simulink model "URDF_XG_Robot_Arm_Urdf_Control_V3"  (R2023a)
settings: Solver=FixedStepAuto  StartTime=0.0  StopTime=20  FixedStep=0.001  RelTol=1e-3
values from neighbouring files (symbols this model uses):
  D_H = [ ... (first row only)    [robot_kinematics_sym_v3_0.m]    (also in robot_kinematics_sym_v3_0_verify.m; robot_run.m)
undefined symbols (not defined in the file or in its folder): X, Y, Z
libraries: sm_lib x62, nesl_utility x11
(part 2 of 2)

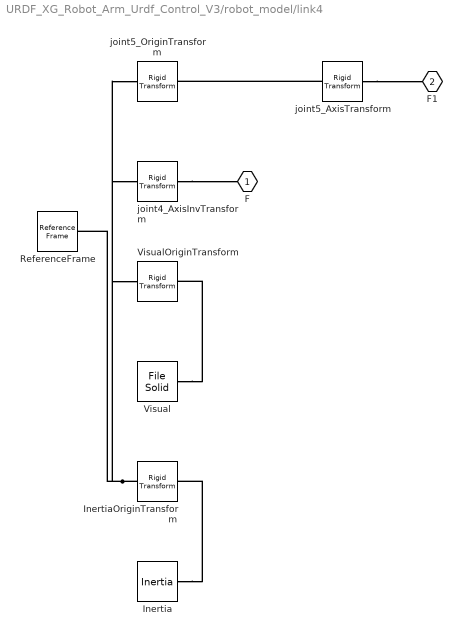
== system URDF_XG_Robot_Arm_Urdf_Control_V3/robot_model/link4 ==
  Inertia : sm_lib/Body Elements/Inertia  InertiaType=Custom  Mass=0.178465854809275  MassUnits=kg  CenterOfMass=[0, 0, 0]  CenterOfMassUnits=m  MomentsOfInertia=[0.00010542070955742, 0.000111293192127703, 4.4231117465552e-05]  MomentsOfInertiaUnits=kg*m^2  ProductsOfInertia=[-4.12005754357462e-07, -1.17627516604833e-07, -1.56493108731347e-07]  ProductsOfInertiaUnits=kg*m^2  GraphicType=None  MarkerShape=Inertia  MarkerSize=20  GraphicVisPropType=SimpleVisualProperties  GraphicDiffuseColor=[0.5 0.5 0.5]  GraphicSpecularColor=[0.5 0.5 0.5 1.0]  GraphicAmbientColor=[0.15 0.15 0.15 1.0]  GraphicEmissiveColor=[0.0 0.0 0.0 1.0]  GraphicShininess=75  GraphicOpacity=1.0
  InertiaOriginTransform : sm_lib/Frames and Transforms/Rigid Transform  TranslationMethod=Cartesian  TranslationStandardOffset=0  TranslationStandardOffsetUnits=m  TranslationStandardAxis=+Z  TranslationCartesianOffset=[-2.8160808468243e-05, -0.00682767077230628, 0.0299455082197141]  TranslationCartesianOffsetUnits=m  TranslationROffset=0  TranslationROffsetUnits=m  TranslationZOffset=0  TranslationZOffsetUnits=m  TranslationThetaOffset=0  TranslationThetaOffsetUnits=deg  RotationMethod=RotationSequence  RotationAngleUnits=deg  RotationStandardAxis=+Z  RotationAngle=0.0  RotationArbitraryAxis=[0 0 1]  FollAlignAxisA=+X  BaseAlignAxisA=+Y  FollAlignAxisB=+Y  BaseAlignAxisB=+Z  RotationSequenceAxes=BaseAxes  RotationSequence=XYZ  RotationSequenceAngles=[0, 0, 0]  RotationSequenceAnglesUnits=rad  RotationMatrix=[1 0 0; 0 1 0; 0 0 1]  Quaternion=[1 0 0 0]
  ReferenceFrame : sm_lib/Frames and Transforms/Reference Frame
  Visual : sm_lib/Body Elements/File Solid  ExtGeomFileName=URDF_XG_Robot_Arm_Urdf_V1_1/meshes/link4.STL  UnitType=Custom  ExtGeomFileUnits=m  StepReaderType=HEX  ExportConvexHullGeometry=off  InertiaType=Custom  Mass=0  MassUnits=kg  CenterOfMass=[0, 0, 0]  CenterOfMassUnits=m  MomentsOfInertia=[0, 0, 0]  MomentsOfInertiaUnits=kg*m^2  ProductsOfInertia=[0, 0, 0]  ProductsOfInertiaUnits=kg*m^2  BasedOnType=DensityFromFile  Density=1000  DensityUnits=kg/m^3  DoExposeReferenceFrame=on  SerializedFrames=<Frames/>  GraphicType=FromGeometry  MarkerShape=Sphere  MarkerSize=10  GraphicVisPropType=SimpleVisualProperties  GraphicDiffuseColor=[0.752941176470588, 0.752941176470588, 0.752941176470588]  GraphicSpecularColor=[0.5 0.5 0.5 1.0]  GraphicAmbientColor=[0.15 0.15 0.15 1.0]  GraphicEmissiveColor=[0.0 0.0 0.0 1.0]  GraphicShininess=75  GraphicOpacity=1
  VisualOriginTransform : sm_lib/Frames and Transforms/Rigid Transform  TranslationMethod=Cartesian  TranslationStandardOffset=0  TranslationStandardOffsetUnits=m  TranslationStandardAxis=+Z  TranslationCartesianOffset=[0, 0, 0]  TranslationCartesianOffsetUnits=m  TranslationROffset=0  TranslationROffsetUnits=m  TranslationZOffset=0  TranslationZOffsetUnits=m  TranslationThetaOffset=0  TranslationThetaOffsetUnits=deg  RotationMethod=RotationSequence  RotationAngleUnits=deg  RotationStandardAxis=+Z  RotationAngle=0.0  RotationArbitraryAxis=[0 0 1]  FollAlignAxisA=+X  BaseAlignAxisA=+Y  FollAlignAxisB=+Y  BaseAlignAxisB=+Z  RotationSequenceAxes=BaseAxes  RotationSequence=XYZ  RotationSequenceAngles=[0, 0, 0]  RotationSequenceAnglesUnits=rad  RotationMatrix=[1 0 0; 0 1 0; 0 0 1]  Quaternion=[1 0 0 0]
  joint4_AxisInvTransform : sm_lib/Frames and Transforms/Rigid Transform  TranslationMethod=Cartesian  TranslationStandardOffset=0  TranslationStandardOffsetUnits=m  TranslationStandardAxis=+Z  TranslationCartesianOffset=[0, 0, 0]  TranslationCartesianOffsetUnits=m  TranslationROffset=0  TranslationROffsetUnits=m  TranslationZOffset=0  TranslationZOffsetUnits=m  TranslationThetaOffset=0  TranslationThetaOffsetUnits=deg  RotationMethod=ArbitraryAxis  RotationAngleUnits=rad  RotationStandardAxis=+Z  RotationAngle=0  RotationArbitraryAxis=[1, 0, 0]  FollAlignAxisA=+X  BaseAlignAxisA=+Y  FollAlignAxisB=+Y  BaseAlignAxisB=+Z  RotationSequenceAxes=FollowerAxes  RotationSequence=XYX  RotationSequenceAngles=[0 0 0]  RotationSequenceAnglesUnits=deg  RotationMatrix=[1 0 0; 0 1 0; 0 0 1]  Quaternion=[1 0 0 0]
  joint5_AxisTransform : sm_lib/Frames and Transforms/Rigid Transform  TranslationMethod=Cartesian  TranslationStandardOffset=0  TranslationStandardOffsetUnits=m  TranslationStandardAxis=+Z  TranslationCartesianOffset=[0, 0, 0]  TranslationCartesianOffsetUnits=m  TranslationROffset=0  TranslationROffsetUnits=m  TranslationZOffset=0  TranslationZOffsetUnits=m  TranslationThetaOffset=0  TranslationThetaOffsetUnits=deg  RotationMethod=ArbitraryAxis  RotationAngleUnits=rad  RotationStandardAxis=+Z  RotationAngle=0  RotationArbitraryAxis=[1, 0, 0]  FollAlignAxisA=+X  BaseAlignAxisA=+Y  FollAlignAxisB=+Y  BaseAlignAxisB=+Z  RotationSequenceAxes=FollowerAxes  RotationSequence=XYX  RotationSequenceAngles=[0 0 0]  RotationSequenceAnglesUnits=deg  RotationMatrix=[1 0 0; 0 1 0; 0 0 1]  Quaternion=[1 0 0 0]
  joint5_OriginTransform : sm_lib/Frames and Transforms/Rigid Transform  TranslationMethod=Cartesian  TranslationStandardOffset=0  TranslationStandardOffsetUnits=m  TranslationStandardAxis=+Z  TranslationCartesianOffset=[0, 0, 0]  TranslationCartesianOffsetUnits=m  TranslationROffset=0  TranslationROffsetUnits=m  TranslationZOffset=0  TranslationZOffsetUnits=m  TranslationThetaOffset=0  TranslationThetaOffsetUnits=deg  RotationMethod=RotationSequence  RotationAngleUnits=deg  RotationStandardAxis=+Z  RotationAngle=0.0  RotationArbitraryAxis=[0 0 1]  FollAlignAxisA=+X  BaseAlignAxisA=+Y  FollAlignAxisB=+Y  BaseAlignAxisB=+Z  RotationSequenceAxes=BaseAxes  RotationSequence=XYZ  RotationSequenceAngles=[1.5708, -1.5708, 0]  RotationSequenceAnglesUnits=rad  RotationMatrix=[1 0 0; 0 1 0; 0 0 1]  Quaternion=[1 0 0 0]
  F : PMIOPort  Side=Left
  F1 : PMIOPort  Port=2  Side=Right
  connections:
  Inertia/RConn1 -- InertiaOriginTransform/RConn1
  ReferenceFrame/RConn1 -- InertiaOriginTransform/LConn1 -- VisualOriginTransform/LConn1 -- joint4_AxisInvTransform/LConn1 -- joint5_OriginTransform/LConn1
  Visual/RConn1 -- VisualOriginTransform/RConn1
  joint4_AxisInvTransform/RConn1 -- F/RConn1
  joint5_AxisTransform/RConn1 -- F1/RConn1
  joint5_AxisTransform/LConn1 -- joint5_OriginTransform/RConn1

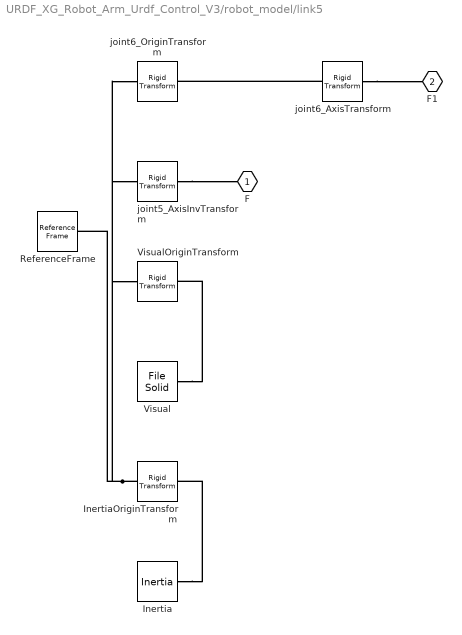
== system URDF_XG_Robot_Arm_Urdf_Control_V3/robot_model/link5 ==
  Inertia : sm_lib/Body Elements/Inertia  InertiaType=Custom  Mass=0.15793222447205  MassUnits=kg  CenterOfMass=[0, 0, 0]  CenterOfMassUnits=m  MomentsOfInertia=[0.000135933655838788, 5.60082572905534e-05, 0.000121456700565665]  MomentsOfInertiaUnits=kg*m^2  ProductsOfInertia=[3.96647905066164e-05, 8.388614449562571e-09, -6.33132038702403e-08]  ProductsOfInertiaUnits=kg*m^2  GraphicType=None  MarkerShape=Inertia  MarkerSize=20  GraphicVisPropType=SimpleVisualProperties  GraphicDiffuseColor=[0.5 0.5 0.5]  GraphicSpecularColor=[0.5 0.5 0.5 1.0]  GraphicAmbientColor=[0.15 0.15 0.15 1.0]  GraphicEmissiveColor=[0.0 0.0 0.0 1.0]  GraphicShininess=75  GraphicOpacity=1.0
  InertiaOriginTransform : sm_lib/Frames and Transforms/Rigid Transform  TranslationMethod=Cartesian  TranslationStandardOffset=0  TranslationStandardOffsetUnits=m  TranslationStandardAxis=+Z  TranslationCartesianOffset=[0.000156431818420899, -0.0617917966301206, -0.0100252833788212]  TranslationCartesianOffsetUnits=m  TranslationROffset=0  TranslationROffsetUnits=m  TranslationZOffset=0  TranslationZOffsetUnits=m  TranslationThetaOffset=0  TranslationThetaOffsetUnits=deg  RotationMethod=RotationSequence  RotationAngleUnits=deg  RotationStandardAxis=+Z  RotationAngle=0.0  RotationArbitraryAxis=[0 0 1]  FollAlignAxisA=+X  BaseAlignAxisA=+Y  FollAlignAxisB=+Y  BaseAlignAxisB=+Z  RotationSequenceAxes=BaseAxes  RotationSequence=XYZ  RotationSequenceAngles=[0, 0, 0]  RotationSequenceAnglesUnits=rad  RotationMatrix=[1 0 0; 0 1 0; 0 0 1]  Quaternion=[1 0 0 0]
  ReferenceFrame : sm_lib/Frames and Transforms/Reference Frame
  Visual : sm_lib/Body Elements/File Solid  ExtGeomFileName=URDF_XG_Robot_Arm_Urdf_V1_1/meshes/link5.STL  UnitType=Custom  ExtGeomFileUnits=m  StepReaderType=HEX  ExportConvexHullGeometry=off  InertiaType=Custom  Mass=0  MassUnits=kg  CenterOfMass=[0, 0, 0]  CenterOfMassUnits=m  MomentsOfInertia=[0, 0, 0]  MomentsOfInertiaUnits=kg*m^2  ProductsOfInertia=[0, 0, 0]  ProductsOfInertiaUnits=kg*m^2  BasedOnType=DensityFromFile  Density=1000  DensityUnits=kg/m^3  DoExposeReferenceFrame=on  SerializedFrames=<Frames/>  GraphicType=FromGeometry  MarkerShape=Sphere  MarkerSize=10  GraphicVisPropType=SimpleVisualProperties  GraphicDiffuseColor=[0.752941176470588, 0.752941176470588, 0.752941176470588]  GraphicSpecularColor=[0.5 0.5 0.5 1.0]  GraphicAmbientColor=[0.15 0.15 0.15 1.0]  GraphicEmissiveColor=[0.0 0.0 0.0 1.0]  GraphicShininess=75  GraphicOpacity=1
  VisualOriginTransform : sm_lib/Frames and Transforms/Rigid Transform  TranslationMethod=Cartesian  TranslationStandardOffset=0  TranslationStandardOffsetUnits=m  TranslationStandardAxis=+Z  TranslationCartesianOffset=[0, 0, 0]  TranslationCartesianOffsetUnits=m  TranslationROffset=0  TranslationROffsetUnits=m  TranslationZOffset=0  TranslationZOffsetUnits=m  TranslationThetaOffset=0  TranslationThetaOffsetUnits=deg  RotationMethod=RotationSequence  RotationAngleUnits=deg  RotationStandardAxis=+Z  RotationAngle=0.0  RotationArbitraryAxis=[0 0 1]  FollAlignAxisA=+X  BaseAlignAxisA=+Y  FollAlignAxisB=+Y  BaseAlignAxisB=+Z  RotationSequenceAxes=BaseAxes  RotationSequence=XYZ  RotationSequenceAngles=[0, 0, 0]  RotationSequenceAnglesUnits=rad  RotationMatrix=[1 0 0; 0 1 0; 0 0 1]  Quaternion=[1 0 0 0]
  joint5_AxisInvTransform : sm_lib/Frames and Transforms/Rigid Transform  TranslationMethod=Cartesian  TranslationStandardOffset=0  TranslationStandardOffsetUnits=m  TranslationStandardAxis=+Z  TranslationCartesianOffset=[0, 0, 0]  TranslationCartesianOffsetUnits=m  TranslationROffset=0  TranslationROffsetUnits=m  TranslationZOffset=0  TranslationZOffsetUnits=m  TranslationThetaOffset=0  TranslationThetaOffsetUnits=deg  RotationMethod=ArbitraryAxis  RotationAngleUnits=rad  RotationStandardAxis=+Z  RotationAngle=0  RotationArbitraryAxis=[1, 0, 0]  FollAlignAxisA=+X  BaseAlignAxisA=+Y  FollAlignAxisB=+Y  BaseAlignAxisB=+Z  RotationSequenceAxes=FollowerAxes  RotationSequence=XYX  RotationSequenceAngles=[0 0 0]  RotationSequenceAnglesUnits=deg  RotationMatrix=[1 0 0; 0 1 0; 0 0 1]  Quaternion=[1 0 0 0]
  joint6_AxisTransform : sm_lib/Frames and Transforms/Rigid Transform  TranslationMethod=Cartesian  TranslationStandardOffset=0  TranslationStandardOffsetUnits=m  TranslationStandardAxis=+Z  TranslationCartesianOffset=[0, 0, 0]  TranslationCartesianOffsetUnits=m  TranslationROffset=0  TranslationROffsetUnits=m  TranslationZOffset=0  TranslationZOffsetUnits=m  TranslationThetaOffset=0  TranslationThetaOffsetUnits=deg  RotationMethod=ArbitraryAxis  RotationAngleUnits=rad  RotationStandardAxis=+Z  RotationAngle=0  RotationArbitraryAxis=[1, 0, 0]  FollAlignAxisA=+X  BaseAlignAxisA=+Y  FollAlignAxisB=+Y  BaseAlignAxisB=+Z  RotationSequenceAxes=FollowerAxes  RotationSequence=XYX  RotationSequenceAngles=[0 0 0]  RotationSequenceAnglesUnits=deg  RotationMatrix=[1 0 0; 0 1 0; 0 0 1]  Quaternion=[1 0 0 0]
  joint6_OriginTransform : sm_lib/Frames and Transforms/Rigid Transform  TranslationMethod=Cartesian  TranslationStandardOffset=0  TranslationStandardOffsetUnits=m  TranslationStandardAxis=+Z  TranslationCartesianOffset=[0, -0.125, 0]  TranslationCartesianOffsetUnits=m  TranslationROffset=0  TranslationROffsetUnits=m  TranslationZOffset=0  TranslationZOffsetUnits=m  TranslationThetaOffset=0  TranslationThetaOffsetUnits=deg  RotationMethod=RotationSequence  RotationAngleUnits=deg  RotationStandardAxis=+Z  RotationAngle=0.0  RotationArbitraryAxis=[0 0 1]  FollAlignAxisA=+X  BaseAlignAxisA=+Y  FollAlignAxisB=+Y  BaseAlignAxisB=+Z  RotationSequenceAxes=BaseAxes  RotationSequence=XYZ  RotationSequenceAngles=[1.5708, 0, 0]  RotationSequenceAnglesUnits=rad  RotationMatrix=[1 0 0; 0 1 0; 0 0 1]  Quaternion=[1 0 0 0]
  F : PMIOPort  Side=Left
  F1 : PMIOPort  Port=2  Side=Right
  connections:
  Inertia/RConn1 -- InertiaOriginTransform/RConn1
  ReferenceFrame/RConn1 -- InertiaOriginTransform/LConn1 -- VisualOriginTransform/LConn1 -- joint5_AxisInvTransform/LConn1 -- joint6_OriginTransform/LConn1
  Visual/RConn1 -- VisualOriginTransform/RConn1
  joint5_AxisInvTransform/RConn1 -- F/RConn1
  joint6_AxisTransform/RConn1 -- F1/RConn1
  joint6_AxisTransform/LConn1 -- joint6_OriginTransform/RConn1

== matlab function URDF_XG_Robot_Arm_Urdf_Control_V3/MATLAB Function1 ==
  data: thetas input; theta output; index input
function theta = theta_selection(thetas, index)

theta = thetas(index, :);

== matlab function URDF_XG_Robot_Arm_Urdf_Control_V3/inv_kinematic/MATLAB Function13 ==
  data: joint_thetas input; thetas_ret output
function thetas_ret = joint_rad2deg(joint_thetas)
thetas_ret = joint_thetas;
for i = 1:4
    for j = 1:6
        thetas_ret(i,j) = rad2deg(thetas_ret(i,j));
    end
end

== matlab function URDF_XG_Robot_Arm_Urdf_Control_V3/inv_kinematic/MATLAB Function1 ==
  data: T_target input; joint_thetas_ret output; joint_thetas input; D_H input
function joint_thetas_ret  = get_theta2(T_target, joint_thetas, D_H)
joint_thetas_ret = zeros(4,6);
joint_thetas_ret(1,:) = joint_thetas(1,:);
joint_thetas_ret(2,:) = joint_thetas(1,:);
joint_thetas_ret(3,:) = joint_thetas(2,:);
joint_thetas_ret(4,:) = joint_thetas(2,:);
joint_thetas_ret(1,2) = get_theta2_1(T_target, joint_thetas_ret(1,3), D_H);
joint_thetas_ret(2,2) = get_theta2_2(T_target, joint_thetas_ret(2,3), D_H);
joint_thetas_ret(3,2) = get_theta2_1(T_target, joint_thetas_ret(3,3), D_H);
joint_thetas_ret(4,2) = get_theta2_2(T_target, joint_thetas_ret(4,3), D_H);
end

function theta2_1 = get_theta2_1(T_target, theta3, D_H)
a_cow = D_H(:, 1);
d_cow = D_H(:, 3);
a2 = a_cow(3);
a3 = a_cow(4);
d4 = d_cow(4);
pz = T_target(3,4);
u1_theta2 = -(a2 + (a2^2 + 2*cos(theta3)*a2*a3 - 2*sin(theta3)*a2*d4 + a3^2 + d4^2 - pz^2)^(1/2) + a3*cos(theta3) - d4*sin(theta3))/(d4*cos(theta3) - pz + a3*sin(theta3));
theta2_1 = atan(u1_theta2)*2;
end

function theta2_2 = get_theta2_2(T_target, theta3, D_H)
a_cow = D_H(:, 1);
d_cow = D_H(:, 3);
a2 = a_cow(3);
a3 = a_cow(4);
d4 = d_cow(4);
pz = T_target(3,4);
u2_theta2 = -(a2 - (a2^2 + 2*cos(theta3)*a2*a3 - 2*sin(theta3)*a2*d4 + a3^2 + d4^2 - pz^2)^(1/2) + a3*cos(theta3) - d4*sin(theta3))/(d4*cos(theta3) - pz + a3*sin(theta3));
theta2_2 = atan(u2_theta2)*2;
end

== matlab function URDF_XG_Robot_Arm_Urdf_Control_V3/inv_kinematic/MATLAB Function ==
  data: T_target input; joint_theatas_ret output; D_H input
function joint_theatas_ret  = get_theta3(T_target, D_H)
a_cow = D_H(:, 1);
d_cow = D_H(:, 3);
a2 = a_cow(3);
a3 = a_cow(4);
d4 = d_cow(4);
px = T_target(1,4);
py = T_target(2,4);
pz = T_target(3,4);
joint_theatas_ret = zeros(2,6);

u1_theta3 = -(2*a2*d4 + (- a2^4 + 2*a2^2*a3^2 + 2*a2^2*d4^2 + 2*a2^2*px^2 + 2*a2^2*py^2 + 2*a2^2*pz^2 - a3^4 - 2*a3^2*d4^2 + 2*a3^2*px^2 + 2*a3^2*py^2 + 2*a3^2*pz^2 - d4^4 + 2*d4^2*px^2 + 2*d4^2*py^2 + 2*d4^2*pz^2 - px^4 - 2*px^2*py^2 - 2*px^2*pz^2 - py^4 - 2*py^2*pz^2 - pz^4)^(1/2))/(- a2^2 + 2*a2*a3 - a3^2 - d4^2 + px^2 + py^2 + pz^2);
u2_theta3 = -(2*a2*d4 - (- a2^4 + 2*a2^2*a3^2 + 2*a2^2*d4^2 + 2*a2^2*px^2 + 2*a2^2*py^2 + 2*a2^2*pz^2 - a3^4 - 2*a3^2*d4^2 + 2*a3^2*px^2 + 2*a3^2*py^2 + 2*a3^2*pz^2 - d4^4 + 2*d4^2*px^2 + 2*d4^2*py^2 + 2*d4^2*pz^2 - px^4 - 2*px^2*py^2 - 2*px^2*pz^2 - py^4 - 2*py^2*pz^2 - pz^4)^(1/2))/(- a2^2 + 2*a2*a3 - a3^2 - d4^2 + px^2 + py^2 + pz^2);
theta3_1 = atan(u1_theta3)*2;
theta3_2 = atan(u2_theta3)*2;
joint_theatas_ret(1, 3) = theta3_1;
joint_theatas_ret(2, 3) = theta3_2;
end

== matlab function URDF_XG_Robot_Arm_Urdf_Control_V3/inv_kinematic/MATLAB Function2 ==
  data: T_target input; joint_thetas output; joint_thetas input; D_H input
function joint_thetas  = get_theta1(T_target, joint_thetas, D_H)
joint_thetas(1,1) = get_theta1_(T_target, joint_thetas(1,:), D_H);
joint_thetas(2,1) = get_theta1_(T_target, joint_thetas(2,:), D_H);
joint_thetas(3,1) = get_theta1_(T_target, joint_thetas(3,:), D_H);
joint_thetas(4,1) = get_theta1_(T_target, joint_thetas(4,:), D_H);
end

function theta1_1 = get_theta1_(T_target, thetas, D_H)
a_cow = D_H(:, 1);
d_cow = D_H(:, 3);
a2 = a_cow(3);
a3 = a_cow(4);
d4 = d_cow(4);
px = T_target(1,4);
py = T_target(2,4);
pz = T_target(3,4);

theta2 = thetas(2);
theta3 = thetas(3);

v1 = (cos(theta2)*(a2 + a3*cos(theta3) - d4*sin(theta3)) + sin(theta2)*(d4*cos(theta3) + a3*sin(theta3)));
v2 = -px/v1;

% 设置容忍度
tolerance = 1e-4;

u1_theta1 = ((v2+1)/(1-v2))^(1/2);
if abs(py - (2*u1_theta1*v1)/(u1_theta1^2 + 1)) > tolerance
    u1_theta1 = -u1_theta1;
end
theta1_1 = atan(u1_theta1)*2;
end

== matlab function URDF_XG_Robot_Arm_Urdf_Control_V3/inv_kinematic/MATLAB Function3 ==
  data: T_target input; joint_thetas_ret output; joint_thetas input; D_H input
function joint_thetas_ret  = get_theta5(T_target, joint_thetas, D_H)
joint_thetas_ret = joint_thetas;
for i = 1:4
    joint_thetas_ret(i, 5) = get_theta5_(T_target, joint_thetas_ret(i, :), D_H);
end
end

function theta5 = get_theta5_(T_target, thetas, D_H)
a_cow = D_H(:, 1);
d_cow = D_H(:, 3);
a2 = a_cow(3);
a3 = a_cow(4);
d4 = d_cow(4);
px = T_target(1,4);
py = T_target(2,4);
pz = T_target(3,4);
nx = T_target(1,1);
ny = T_target(2,1);
nz = T_target(3,1);
ox = T_target(1,2);
oy = T_target(2,2);
oz = T_target(3,2);
ax= T_target(1,3);
ay= T_target(2,3);
az= T_target(3,3);
theta2 = thetas(2);
theta3 = thetas(3);
theta1 = thetas(1);

r32 = - (oz*(cos(theta2)*cos(theta3) + sin(theta2)*sin(theta3)))/(cos(theta2)^2*cos(theta3)^2 + cos(theta2)^2*sin(theta3)^2 + cos(theta3)^2*sin(theta2)^2 + sin(theta2)^2*sin(theta3)^2) - (ox*(cos(theta1)*cos(theta2)*sin(theta3) - cos(theta1)*cos(theta3)*sin(theta2)))/(cos(theta1)^2*cos(theta2)^2*cos(theta3)^2 + cos(theta1)^2*cos(theta2)^2*sin(theta3)^2 + cos(theta1)^2*cos(theta3)^2*sin(theta2)^2 + cos(theta1)^2*sin(theta2)^2*sin(theta3)^2 + cos(theta2)^2*cos(theta3)^2*sin(theta1)^2 + cos(theta2)^2*sin(theta1)^2*sin(theta3)^2 + cos(theta3)^2*sin(theta1)^2*sin(theta2)^2 + sin(theta1)^2*sin(theta2)^2*sin(theta3)^2) - (oy*(cos(theta2)*sin(theta1)*sin(theta3) - cos(theta3)*sin(theta1)*sin(theta2)))/(cos(theta1)^2*cos(theta2)^2*cos(theta3)^2 + cos(theta1)^2*cos(theta2)^2*sin(theta3)^2 + cos(theta1)^2*cos(theta3)^2*sin(theta2)^2 + cos(theta1)^2*sin(theta2)^2*sin(theta3)^2 + cos(theta2)^2*cos(theta3)^2*sin(theta1)^2 + cos(theta2)^2*sin(theta1)^2*sin(theta3)^2 + cos(theta3)^2*sin(theta1)^2*sin(theta2)^2 + sin(theta1)^2*sin(theta2)^2*sin(theta3)^2);
r31 = - (nz*(cos(theta2)*cos(theta3) + sin(theta2)*sin(theta3)))/(cos(theta2)^2*cos(theta3)^2 + cos(theta2)^2*sin(theta3)^2 + cos(theta3)^2*sin(theta2)^2 + sin(theta2)^2*sin(theta3)^2) - (nx*(cos(theta1)*cos(theta2)*sin(theta3) - cos(theta1)*cos(theta3)*sin(theta2)))/(cos(theta1)^2*cos(theta2)^2*cos(theta3)^2 + cos(theta1)^2*cos(theta2)^2*sin(theta3)^2 + cos(theta1)^2*cos(theta3)^2*sin(theta2)^2 + cos(theta1)^2*sin(theta2)^2*sin(theta3)^2 + cos(theta2)^2*cos(theta3)^2*sin(theta1)^2 + cos(theta2)^2*sin(theta1)^2*sin(theta3)^2 + cos(theta3)^2*sin(theta1)^2*sin(theta2)^2 + sin(theta1)^2*sin(theta2)^2*sin(theta3)^2) - (ny*(cos(theta2)*sin(theta1)*sin(theta3) - cos(theta3)*sin(theta1)*sin(theta2)))/(cos(theta1)^2*cos(theta2)^2*cos(theta3)^2 + cos(theta1)^2*cos(theta2)^2*sin(theta3)^2 + cos(theta1)^2*cos(theta3)^2*sin(theta2)^2 + cos(theta1)^2*sin(theta2)^2*sin(theta3)^2 + cos(theta2)^2*cos(theta3)^2*sin(theta1)^2 + cos(theta2)^2*sin(theta1)^2*sin(theta3)^2 + cos(theta3)^2*sin(theta1)^2*sin(theta2)^2 + sin(theta1)^2*sin(theta2)^2*sin(theta3)^2);
r33 = - (az*(cos(theta2)*cos(theta3) + sin(theta2)*sin(theta3)))/(cos(theta2)^2*cos(theta3)^2 + cos(theta2)^2*sin(theta3)^2 + cos(theta3)^2*sin(theta2)^2 + sin(theta2)^2*sin(theta3)^2) - (ax*(cos(theta1)*cos(theta2)*sin(theta3) - cos(theta1)*cos(theta3)*sin(theta2)))/(cos(theta1)^2*cos(theta2)^2*cos(theta3)^2 + cos(theta1)^2*cos(theta2)^2*sin(theta3)^2 + cos(theta1)^2*cos(theta3)^2*sin(theta2)^2 + cos(theta1)^2*sin(theta2)^2*sin(theta3)^2 + cos(theta2)^2*cos(theta3)^2*sin(theta1)^2 + cos(theta2)^2*sin(theta1)^2*sin(theta3)^2 + cos(theta3)^2*sin(theta1)^2*sin(theta2)^2 + sin(theta1)^2*sin(theta2)^2*sin(theta3)^2) - (ay*(cos(theta2)*sin(theta1)*sin(theta3) - cos(theta3)*sin(theta1)*sin(theta2)))/(cos(theta1)^2*cos(theta2)^2*cos(theta3)^2 + cos(theta1)^2*cos(theta2)^2*sin(theta3)^2 + cos(theta1)^2*cos(theta3)^2*sin(theta2)^2 + cos(theta1)^2*sin(theta2)^2*sin(theta3)^2 + cos(theta2)^2*cos(theta3)^2*sin(theta1)^2 + cos(theta2)^2*sin(theta1)^2*sin(theta3)^2 + cos(theta3)^2*sin(theta1)^2*sin(theta2)^2 + sin(theta1)^2*sin(theta2)^2*sin(theta3)^2);
theta5 = atan2(sqrt(r32^2 + r31^2), r33);
theta5 = -theta5 + pi;
end

== matlab function URDF_XG_Robot_Arm_Urdf_Control_V3/inv_kinematic/MATLAB Function4 ==
  data: T_target input; joint_thetas_ret output; joint_thetas input; D_H input
function joint_thetas_ret  = get_theta4(T_target, joint_thetas, D_H)
joint_thetas_ret = joint_thetas;
for i = 1:4
    joint_thetas_ret(i, 4) = get_theta4_(T_target, joint_thetas_ret(i, :), D_H);
end
end

function theta4_value = get_theta4_(T_target, thetas, D_H)
% deg_theta5_zyz = rad2deg(-thetas(5) + pi);
% if deg_theta5_zyz == 0 || deg_theta5_zyz == 180
%     theta4_value = 0;
%     return;
% end
a_cow = D_H(:, 1);
d_cow = D_H(:, 3);
a2 = a_cow(3);
a3 = a_cow(4);
d4 = d_cow(4);
px = T_target(1,4);
py = T_target(2,4);
pz = T_target(3,4);
nx = T_target(1,1);
ny = T_target(2,1);
nz = T_target(3,1);
ox = T_target(1,2);
oy = T_target(2,2);
oz = T_target(3,2);
ax= T_target(1,3);
ay= T_target(2,3);
az= T_target(3,3);
theta2 = thetas(2);
theta3 = thetas(3);
theta1 = thetas(1);
theta4 = 0; % 这里特殊，用于坐标系对齐
r23 = -(ax*cos(theta1)*cos(theta2)*cos(theta3)*sin(theta4) - ax*cos(theta4)*sin(theta1)*sin(theta2)^2*sin(theta3)^2 + ay*cos(theta2)*cos(theta3)*sin(theta1)*sin(theta4) + ax*cos(theta1)*sin(theta2)*sin(theta3)*sin(theta4) + ay*sin(theta1)*sin(theta2)*sin(theta3)*sin(theta4) - az*cos(theta1)^2*cos(theta2)*sin(theta3)*sin(theta4) + az*cos(theta1)^2*cos(theta3)*sin(theta2)*sin(theta4) - az*cos(theta2)*sin(theta1)^2*sin(theta3)*sin(theta4) + az*cos(theta3)*sin(theta1)^2*sin(theta2)*sin(theta4) + ay*cos(theta1)*cos(theta2)^2*cos(theta3)^2*cos(theta4) - ax*cos(theta2)^2*cos(theta3)^2*cos(theta4)*sin(theta1) + ay*cos(theta1)*cos(theta2)^2*cos(theta4)*sin(theta3)^2 + ay*cos(theta1)*cos(theta3)^2*cos(theta4)*sin(theta2)^2 - ax*cos(theta2)^2*cos(theta4)*sin(theta1)*sin(theta3)^2 - ax*cos(theta3)^2*cos(theta4)*sin(theta1)*sin(theta2)^2 + ay*cos(theta1)*cos(theta4)*sin(theta2)^2*sin(theta3)^2)/((cos(theta1)^2*cos(theta4)^2 + cos(theta1)^2*sin(theta4)^2 + cos(theta4)^2*sin(theta1)^2 + sin(theta1)^2*sin(theta4)^2)*(cos(theta2)^2*cos(theta3)^2 + cos(theta2)^2*sin(theta3)^2 + cos(theta3)^2*sin(theta2)^2 + sin(theta2)^2*sin(theta3)^2));
r13 = (-az*cos(theta4)*cos(theta1)^2*cos(theta2)*sin(theta3) + az*cos(theta4)*cos(theta1)^2*cos(theta3)*sin(theta2) - ay*sin(theta4)*cos(theta1)*cos(theta2)^2*cos(theta3)^2 - ay*sin(theta4)*cos(theta1)*cos(theta2)^2*sin(theta3)^2 + ax*cos(theta4)*cos(theta1)*cos(theta2)*cos(theta3) - ay*sin(theta4)*cos(theta1)*cos(theta3)^2*sin(theta2)^2 - ay*sin(theta4)*cos(theta1)*sin(theta2)^2*sin(theta3)^2 + ax*cos(theta4)*cos(theta1)*sin(theta2)*sin(theta3) + ax*sin(theta4)*cos(theta2)^2*cos(theta3)^2*sin(theta1) + ax*sin(theta4)*cos(theta2)^2*sin(theta1)*sin(theta3)^2 + ay*cos(theta4)*cos(theta2)*cos(theta3)*sin(theta1) - az*cos(theta4)*cos(theta2)*sin(theta1)^2*sin(theta3) + ax*sin(theta4)*cos(theta3)^2*sin(theta1)*sin(theta2)^2 + az*cos(theta4)*cos(theta3)*sin(theta1)^2*sin(theta2) + ax*sin(theta4)*sin(theta1)*sin(theta2)^2*sin(theta3)^2 + ay*cos(theta4)*sin(theta1)*sin(theta2)*sin(theta3))/((cos(theta1)^2 + sin(theta1)^2)*(cos(theta4)^2 + sin(theta4)^2)*(cos(theta2)^2*cos(theta3)^2 + cos(theta2)^2*sin(theta3)^2 + cos(theta3)^2*sin(theta2)^2 + sin(theta2)^2*sin(theta3)^2));
theta4_value = atan2(r23, r13);
end

== matlab function URDF_XG_Robot_Arm_Urdf_Control_V3/inv_kinematic/MATLAB Function5 ==
  data: T_target input; joint_thetas_ret output; joint_thetas input; D_H input
function joint_thetas_ret  = get_theta6(T_target, joint_thetas, D_H)
joint_thetas_ret = joint_thetas;
for i = 1:4
    joint_thetas_ret(i, 6) = get_theta6_(T_target, joint_thetas_ret(i, :), D_H);
end
end

function theta6_value = get_theta6_(T_target, thetas, D_H)
a_cow = D_H(:, 1);
d_cow = D_H(:, 3);
a2 = a_cow(3);
a3 = a_cow(4);
d4 = d_cow(4);
px = T_target(1,4);
py = T_target(2,4);
pz = T_target(3,4);
nx = T_target(1,1);
ny = T_target(2,1);
nz = T_target(3,1);
ox = T_target(1,2);
oy = T_target(2,2);
oz = T_target(3,2);
ax= T_target(1,3);
ay= T_target(2,3);
az= T_target(3,3);
theta2 = thetas(2);
theta3 = thetas(3);
theta1 = thetas(1);
theta4 = 0;
% deg_theta5_zyz = rad2deg(-thetas(5) + pi);
% if deg_theta5_zyz == 0 || deg_theta5_zyz == 180
%     r12 = (ox*(sin(theta1)*sin(theta4)*cos(theta2)^2*cos(theta3)^2 + sin(theta1)*sin(theta4)*cos(theta2)^2*sin(theta3)^2 + cos(theta1)*cos(theta4)*cos(theta2)*cos(theta3) + sin(theta1)*sin(theta4)*cos(theta3)^2*sin(theta2)^2 + sin(theta1)*sin(theta4)*sin(theta2)^2*sin(theta3)^2 + cos(theta1)*cos(theta4)*sin(theta2)*sin(theta3)))/(cos(theta1)^2*cos(theta2)^2*cos(theta3)^2*cos(theta4)^2 + cos(theta1)^2*cos(theta2)^2*cos(theta3)^2*sin(theta4)^2 + cos(theta1)^2*cos(theta2)^2*cos(theta4)^2*sin(theta3)^2 + cos(theta1)^2*cos(theta2)^2*sin(theta3)^2*sin(theta4)^2 + cos(theta1)^2*cos(theta3)^2*cos(theta4)^2*sin(theta2)^2 + cos(theta1)^2*cos(theta3)^2*sin(theta2)^2*sin(theta4)^2 + cos(theta1)^2*cos(theta4)^2*sin(theta2)^2*sin(theta3)^2 + cos(theta1)^2*sin(theta2)^2*sin(theta3)^2*sin(theta4)^2 + cos(theta2)^2*cos(theta3)^2*cos(theta4)^2*sin(theta1)^2 + cos(theta2)^2*cos(theta3)^2*sin(theta1)^2*sin(theta4)^2 + cos(theta2)^2*cos(theta4)^2*sin(theta1)^2*sin(theta3)^2 + cos(theta2)^2*sin(theta1)^2*sin(theta3)^2*sin(theta4)^2 + cos(theta3)^2*cos(theta4)^2*sin(theta1)^2*sin(theta2)^2 + cos(theta3)^2*sin(theta1)^2*sin(theta2)^2*sin(theta4)^2 + cos(theta4)^2*sin(theta1)^2*sin(theta2)^2*sin(theta3)^2 + sin(theta1)^2*sin(theta2)^2*sin(theta3)^2*sin(theta4)^2) - (oz*(cos(theta2)*cos(theta4)*sin(theta3) - cos(theta3)*cos(theta4)*sin(theta2)))/(cos(theta2)^2*cos(theta3)^2*cos(theta4)^2 + cos(theta2)^2*cos(theta3)^2*sin(theta4)^2 + cos(theta2)^2*cos(theta4)^2*sin(theta3)^2 + cos(theta2)^2*sin(theta3)^2*sin(theta4)^2 + cos(theta3)^2*cos(theta4)^2*sin(theta2)^2 + cos(theta3)^2*sin(theta2)^2*sin(theta4)^2 + cos(theta4)^2*sin(theta2)^2*sin(theta3)^2 + sin(theta2)^2*sin(theta3)^2*sin(theta4)^2) - (oy*(cos(theta1)*sin(theta4)*cos(theta2)^2*cos(theta3)^2 + cos(theta1)*sin(theta4)*cos(theta2)^2*sin(theta3)^2 - cos(theta4)*sin(theta1)*cos(theta2)*cos(theta3) + cos(theta1)*sin(theta4)*cos(theta3)^2*sin(theta2)^2 + cos(theta1)*sin(theta4)*sin(theta2)^2*sin(theta3)^2 - cos(theta4)*sin(theta1)*sin(theta2)*sin(theta3)))/(cos(theta1)^2*cos(theta2)^2*cos(theta3)^2*cos(theta4)^2 + cos(theta1)^2*cos(theta2)^2*cos(theta3)^2*sin(theta4)^2 + cos(theta1)^2*cos(theta2)^2*cos(theta4)^2*sin(theta3)^2 + cos(theta1)^2*cos(theta2)^2*sin(theta3)^2*sin(theta4)^2 + cos(theta1)^2*cos(theta3)^2*cos(theta4)^2*sin(theta2)^2 + cos(theta1)^2*cos(theta3)^2*sin(theta2)^2*sin(theta4)^2 + cos(theta1)^2*cos(theta4)^2*sin(theta2)^2*sin(theta3)^2 + cos(theta1)^2*sin(theta2)^2*sin(theta3)^2*sin(theta4)^2 + cos(theta2)^2*cos(theta3)^2*cos(theta4)^2*sin(theta1)^2 + cos(theta2)^2*cos(theta3)^2*sin(theta1)^2*sin(theta4)^2 + cos(theta2)^2*cos(theta4)^2*sin(theta1)^2*sin(theta3)^2 + cos(theta2)^2*sin(theta1)^2*sin(theta3)^2*sin(theta4)^2 + cos(theta3)^2*cos(theta4)^2*sin(theta1)^2*sin(theta2)^2 + cos(theta3)^2*sin(theta1)^2*sin(theta2)^2*sin(theta4)^2 + cos(theta4)^2*sin(theta1)^2*sin(theta2)^2*sin(theta3)^2 + sin(theta1)^2*sin(theta2)^2*sin(theta3)^2*sin(theta4)^2);
%     r11 = (nx*(sin(theta1)*sin(theta4)*cos(theta2)^2*cos(theta3)^2 + sin(theta1)*sin(theta4)*cos(theta2)^2*sin(theta3)^2 + cos(theta1)*cos(theta4)*cos(theta2)*cos(theta3) + sin(theta1)*sin(theta4)*cos(theta3)^2*sin(theta2)^2 + sin(theta1)*sin(theta4)*sin(theta2)^2*sin(theta3)^2 + cos(theta1)*cos(theta4)*sin(theta2)*sin(theta3)))/(cos(theta1)^2*cos(theta2)^2*cos(theta3)^2*cos(theta4)^2 + cos(theta1)^2*cos(theta2)^2*cos(theta3)^2*sin(theta4)^2 + cos(theta1)^2*cos(theta2)^2*cos(theta4)^2*sin(theta3)^2 + cos(theta1)^2*cos(theta2)^2*sin(theta3)^2*sin(theta4)^2 + cos(theta1)^2*cos(theta3)^2*cos(theta4)^2*sin(theta2)^2 + cos(theta1)^2*cos(theta3)^2*sin(theta2)^2*sin(theta4)^2 + cos(theta1)^2*cos(theta4)^2*sin(theta2)^2*sin(theta3)^2 + cos(theta1)^2*sin(theta2)^2*sin(theta3)^2*sin(theta4)^2 + cos(theta2)^2*cos(theta3)^2*cos(theta4)^2*sin(theta1)^2 + cos(theta2)^2*cos(theta3)^2*sin(theta1)^2*sin(theta4)^2 + cos(theta2)^2*cos(theta4)^2*sin(theta1)^2*sin(theta3)^2 + cos(theta2)^2*sin(theta1)^2*sin(theta3)^2*sin(theta4)^2 + cos(theta3)^2*cos(theta4)^2*sin(theta1)^2*sin(theta2)^2 + cos(theta3)^2*sin(theta1)^2*sin(theta2)^2*sin(theta4)^2 + cos(theta4)^2*sin(theta1)^2*sin(theta2)^2*sin(theta3)^2 + sin(theta1)^2*sin(theta2)^2*sin(theta3)^2*sin(theta4)^2) - (nz*(cos(theta2)*cos(theta4)*sin(theta3) - cos(theta3)*cos(theta4)*sin(theta2)))/(cos(theta2)^2*cos(theta3)^2*cos(theta4)^2 + cos(theta2)^2*cos(theta3)^2*sin(theta4)^2 + cos(theta2)^2*cos(theta4)^2*sin(theta3)^2 + cos(theta2)^2*sin(theta3)^2*sin(theta4)^2 + cos(theta3)^2*cos(theta4)^2*sin(theta2)^2 + cos(theta3)^2*sin(theta2)^2*sin(theta4)^2 + cos(theta4)^2*sin(theta2)^2*sin(theta3)^2 + sin(theta2)^2*sin(theta3)^2*sin(theta4)^2) - (ny*(cos(theta1)*sin(theta4)*cos(theta2)^2*cos(theta3)^2 + cos(theta1)*sin(theta4)*cos(theta2)^2*sin(theta3)^2 - cos(theta4)*sin(theta1)*cos(theta2)*cos(theta3) + cos(theta1)*sin(theta4)*cos(theta3)^2*sin(theta2)^2 + cos(theta1)*sin(theta4)*sin(theta2)^2*sin(theta3)^2 - cos(theta4)*sin(theta1)*sin(theta2)*sin(theta3)))/(cos(theta1)^2*cos(theta2)^2*cos(theta3)^2*cos(theta4)^2 + cos(theta1)^2*cos(theta2)^2*cos(theta3)^2*sin(theta4)^2 + cos(theta1)^2*cos(theta2)^2*cos(theta4)^2*sin(theta3)^2 + cos(theta1)^2*cos(theta2)^2*sin(theta3)^2*sin(theta4)^2 + cos(theta1)^2*cos(theta3)^2*cos(theta4)^2*sin(theta2)^2 + cos(theta1)^2*cos(theta3)^2*sin(theta2)^2*sin(theta4)^2 + cos(theta1)^2*cos(theta4)^2*sin(theta2)^2*sin(theta3)^2 + cos(theta1)^2*sin(theta2)^2*sin(theta3)^2*sin(theta4)^2 + cos(theta2)^2*cos(theta3)^2*cos(theta4)^2*sin(theta1)^2 + cos(theta2)^2*cos(theta3)^2*sin(theta1)^2*sin(theta4)^2 + cos(theta2)^2*cos(theta4)^2*sin(theta1)^2*sin(theta3)^2 + cos(theta2)^2*sin(theta1)^2*sin(theta3)^2*sin(theta4)^2 + cos(theta3)^2*cos(theta4)^2*sin(theta1)^2*sin(theta2)^2 + cos(theta3)^2*sin(theta1)^2*sin(theta2)^2*sin(theta4)^2 + cos(theta4)^2*sin(theta1)^2*sin(theta2)^2*sin(theta3)^2 + sin(theta1)^2*sin(theta2)^2*sin(theta3)^2*sin(theta4)^2);
%     theta6_value = atan2(-r12, r11);
%     theta6_value = theta6_value - pi;
%     return;
% end

r32 = - (oz*(cos(theta2)*cos(theta3) + sin(theta2)*sin(theta3)))/(cos(theta2)^2*cos(theta3)^2 + cos(theta2)^2*sin(theta3)^2 + cos(theta3)^2*sin(theta2)^2 + sin(theta2)^2*sin(theta3)^2) - (ox*(cos(theta1)*cos(theta2)*sin(theta3) - cos(theta1)*cos(theta3)*sin(theta2)))/(cos(theta1)^2*cos(theta2)^2*cos(theta3)^2 + cos(theta1)^2*cos(theta2)^2*sin(theta3)^2 + cos(theta1)^2*cos(theta3)^2*sin(theta2)^2 + cos(theta1)^2*sin(theta2)^2*sin(theta3)^2 + cos(theta2)^2*cos(theta3)^2*sin(theta1)^2 + cos(theta2)^2*sin(theta1)^2*sin(theta3)^2 + cos(theta3)^2*sin(theta1)^2*sin(theta2)^2 + sin(theta1)^2*sin(theta2)^2*sin(theta3)^2) - (oy*(cos(theta2)*sin(theta1)*sin(theta3) - cos(theta3)*sin(theta1)*sin(theta2)))/(cos(theta1)^2*cos(theta2)^2*cos(theta3)^2 + cos(theta1)^2*cos(theta2)^2*sin(theta3)^2 + cos(theta1)^2*cos(theta3)^2*sin(theta2)^2 + cos(theta1)^2*sin(theta2)^2*sin(theta3)^2 + cos(theta2)^2*cos(theta3)^2*sin(theta1)^2 + cos(theta2)^2*sin(theta1)^2*sin(theta3)^2 + cos(theta3)^2*sin(theta1)^2*sin(theta2)^2 + sin(theta1)^2*sin(theta2)^2*sin(theta3)^2);
r31 = - (nz*(cos(theta2)*cos(theta3) + sin(theta2)*sin(theta3)))/(cos(theta2)^2*cos(theta3)^2 + cos(theta2)^2*sin(theta3)^2 + cos(theta3)^2*sin(theta2)^2 + sin(theta2)^2*sin(theta3)^2) - (nx*(cos(theta1)*cos(theta2)*sin(theta3) - cos(theta1)*cos(theta3)*sin(theta2)))/(cos(theta1)^2*cos(theta2)^2*cos(theta3)^2 + cos(theta1)^2*cos(theta2)^2*sin(theta3)^2 + cos(theta1)^2*cos(theta3)^2*sin(theta2)^2 + cos(theta1)^2*sin(theta2)^2*sin(theta3)^2 + cos(theta2)^2*cos(theta3)^2*sin(theta1)^2 + cos(theta2)^2*sin(theta1)^2*sin(theta3)^2 + cos(theta3)^2*sin(theta1)^2*sin(theta2)^2 + sin(theta1)^2*sin(theta2)^2*sin(theta3)^2) - (ny*(cos(theta2)*sin(theta1)*sin(theta3) - cos(theta3)*sin(theta1)*sin(theta2)))/(cos(theta1)^2*cos(theta2)^2*cos(theta3)^2 + cos(theta1)^2*cos(theta2)^2*sin(theta3)^2 + cos(theta1)^2*cos(theta3)^2*sin(theta2)^2 + cos(theta1)^2*sin(theta2)^2*sin(theta3)^2 + cos(theta2)^2*cos(theta3)^2*sin(theta1)^2 + cos(theta2)^2*sin(theta1)^2*sin(theta3)^2 + cos(theta3)^2*sin(theta1)^2*sin(theta2)^2 + sin(theta1)^2*sin(theta2)^2*sin(theta3)^2);
theta6_value = atan2(r32, -r31);
theta6_value = theta6_value - pi;
end

== matlab function URDF_XG_Robot_Arm_Urdf_Control_V3/inv_kinematic/MATLAB Function6 ==
  data: joint_thetas input; D_H input; theta_ret output; thetas output; theta_diffs output; best_diff_index output
function [theta_ret, thetas, theta_diffs, best_diff_index]  = get_best_joint_theta(joint_thetas, D_H)
% theta_ret: 最优一组的关节相对于初始位置的旋转角度
% thetas: 所有组的关节相对于初始位置的旋转角度
% theta_diffs：所有组的与当前关节角度变化的绝对值总和，即与当前位置的差异，其大小表示需要变化的难度
thetas = joint_thetas;
    theta_diffs = zeros(1,4);
    persistent current_theta
    if isempty(current_theta)
        current_theta = zeros(1,6);
    end

    for i = 1:4
        [theta, theta_diff] = joint_theta_change(thetas(i, :), current_theta, D_H);
        thetas(i, :) = theta;
        theta_diffs(i) = theta_diff;
    end
    [~, best_diff_index] = min(theta_diffs);
    theta_ret = thetas(best_diff_index, :);
    current_theta = theta_ret;
end

function [theta_ret, theta_diff] = joint_theta_change(theta, current_theta, D_H)
    % theta_diff: 与当前关节角度变化的绝对值总和，即与当前位置的差异，其大小表示需要变化的难度
    theta_ret = zeros(1,6);
    theta_diff = 0;
    for i = 1:6
        tmp_theta = mod(theta(i) + 360, 360);
        init_theta = mod(rad2deg(D_H(i, 4)) + 360, 360);
        theta_ret(i) = tmp_theta - init_theta;
        theta_diff = theta_diff + (7 - i) * abs(theta_ret(i) - current_theta(i)); % 与当前位置的差异
    end
end

== matlab function URDF_XG_Robot_Arm_Urdf_Control_V3/MATLAB Function ==
  data: xyz input; T_target output; rot input
function T_target = T_target_genrate(xyz, rot)
T_target = [rot xyz; 0 0 0 1];

== matlab function URDF_XG_Robot_Arm_Urdf_Control_V3/kinematics/MATLAB Function ==
  data: D_H input; T0_1 output; T1_2 output; T2_3 output; T3_4 output; T4_5 output; T5_6 output; joints_theata input; T0_6 output
function [T0_1, T1_2, T2_3, T3_4, T4_5, T5_6, T0_6] = get_links_trans(D_H, joints_theata)
% 获得连杆变化矩阵
% D_H: D-H表
% joints_theta: 当前各关节角度 rad
T0_1 = get_link_trans(D_H(1,:), joints_theata(1));
T1_2 = get_link_trans(D_H(2,:), joints_theata(2));
T2_3 = get_link_trans(D_H(3,:), joints_theata(3));
T3_4 = get_link_trans(D_H(4,:), joints_theata(4));
T4_5 = get_link_trans(D_H(5,:), joints_theata(5));
T5_6 = get_link_trans(D_H(6,:), joints_theata(6));
T0_6 = T0_1 * T1_2 * T2_3 * T3_4 * T4_5 * T5_6;
end

function T = get_link_trans(D_H_link, joint_theta)
a = D_H_link(1);
alpha = D_H_link(2);
d = D_H_link(3);
theta = joint_theta;
T = [cos(theta), -sin(theta), 0, a;
    sin(theta)*cos(alpha), cos(theta)*cos(alpha), -sin(alpha), -d*sin(alpha);
    sin(theta)*sin(alpha), cos(theta)*sin(alpha), cos(alpha), d*cos(alpha);
    0, 0, 0, 1];
end
